simulink model "VehCtrl20260630_18B"  (R2018b)
settings: Solver=FixedStepAuto  StartTime=0.0  StopTime=inf  FixedStep=0.005  RelTol=1e-3
InitFcn:
  | mbd_mpc_consistency_checks(bdroot(gcs));
undefined symbols (not defined in the file): ANG_DEAD, BMS_NormalPwr, BrakeDeadZone, BrkPrsByBrkPct_TB_X, BrkPrsByBrkPct_TB_Y, DELAY_DISCHARGE, DELAY_RCUOFF, DRV_BACKWARD, DRV_BRAKE, DRV_FORWARD, DRV_NEUTRAL, DRV_PARK, DRV_UNPARK, DRV_ZEROTURN, EPB_LOCK, EPB_UNLOCK, ExtraLoadPwr, FanOff, fifo_0_vect, fifo_1_vect, HiFanReq, HV_finished, HV_No_Active, HV_POWER_OFF, HV_POWER_ON, HVDown, HVON, KaTLS_v_DrgUp_X_VehSpd, KeFTM_s_Way1OffDlyTime, KeFTM_TK_Way1CoolLv2OffBatTemp, KeFTM_TK_Way1CoolLv2OffMtrTemp, KeFTM_TK_Way1CoolLv2OnBatTemp, KeFTM_TK_Way1CoolLv2OnMtrTemp, KeFTM_TK_Way1CoolLv3OffBatTemp, KeFTM_TK_Way1CoolLv3OffMtrTemp, KeFTM_TK_Way1CoolLv3OnBatTemp, KeFTM_TK_Way1CoolLv3OnMtrTemp, KeFTM_TK_Way1CoolLv4OffBatTemp, KeFTM_TK_Way1CoolLv4OffMtrTemp, KeFTM_TK_Way1CoolLv4OnBatTemp, KeFTM_TK_Way1CoolLv4OnMtrTemp, Kp1, Kp2, LowFanReq, LQFP, MtrCmdGainFL, MtrCmdGainFR, MtrCmdGainRL, MtrCmdGainRR, MtrPwrFactor_RCU, MtrPwrHighToMidThd, MtrPwrLowToMidThd, MtrPwrMidToHighThd, MtrPwrMidToLowThd, MtrTrqMax, PCT_DEAD, Precharge, PTO_1000, PTO_540, pts1_fifo_0_vect ... (+32)
libraries: mbd_mpc574x_ec_toolbox x175, simulink x110, canmsglib x70
(part 14 of 15)

== system VehCtrl20260630_18B/SigIn/CAN0/AUTO2/UNPACK/Subsystem ==
  In1 : Inport
  CAN_Msg_In : Inport  Port=2
  Action Port : ActionPort  ActionType=else
  Bus Creator1 : BusCreator  Inputs=9
  CAN Unpack6 : canmsglib/CAN Unpack  CANdbFile=E:\硕士工作\0.本周工作\20260428_changchun\VCU_AgriculturalMachinery_260428_ChangChun\VCU_AgriculturalMachinery_260428_ChangChun\CAN协议9.1\AUTO\TractorAuto_Intel.dbc  MsgList=AUTO2VCU_2  MsgName=AUTO2VCU_2  MsgIDType=Extended (29-bit identifier)  MsgIdentifier=4098  MsgLength=8  SignalInfo=AUTO_CheckSum2$56$8$1$2$1$0$1$0$0$255$#AUTO_LiveCnt2$52$4$1$2$1$0$1$0$0$15$#AUTO_PtoSpd$0$16$1$2$1$0$1.000000e-01$-3000$-3000$3000$#AUTO_Shutdown$18$1$1$2$1$0$1$0$0$1$#AUTO_SuspMode$16$2$1$2$1$0$1$0$0$3$#AUTO_Valve1$19$1$1$2$1$0$1$0$0$1$#AUTO_Valve2$20$1$1$2$1$0$1$0$0$1$#AUTO_Valve3$21$1$1$2$1$0$1$0$0$1$#AUTO_Valve4$22$1$1$2$1$0$1$0$0$1$#  NSignals=9  IDPort=off  TimestampPort=off  ErrorPort=off  RemotePort=off  LengthPort=off  StatusPort=off  StartBits=str2num('[int32(56);int32(52);int32(0);int32(18);int32(16);int32(19);int32(20);int32(21);int32(22)]')  SignalSizes=str2num('[int32(8);int32(4);int32(16);int32(1);int32(2);int32(1);int32(1);int32(1);int32(1)]')  ByteOrders=str2num('[int32(1);int32(1);int32(1);int32(1);int32(1);int32(1);int32(1);int32(1);int32(1)]')  DataTypes=str2num('[int32(2);int32(2);int32(2);int32(2);int32(2);int32(2);int32(2);int32(2);int32(2)]')  MultiplexTypes=str2num('[int32(1);int32(1);int32(1);int32(1);int32(1);int32(1);int32(1);int32(1);int32(1)]')  MultiplexValues=str2num('[double(0);double(0);double(0);double(0);double(0);double(0);double(0);double(0);double(0)]')  Factors=str2num('[double(1);double(1);double(1.000000e-01);double(1);double(1);double(1);double(1);double(1);double(1)]')  Offsets=str2num('[double(0);double(0);double(-3000);double(0);double(0);double(0);double(0);double(0);double(0)]')  Minimums=str2num('[double(0);double(0);double(-3000);double(0);double(0);double(0);double(0);double(0);double(0)]')  Maximums=str2num('[double(255);double(15);double(3000);double(1);double(3);double(1);double(1);double(1);double(1)]')  ApplyMinMax=off
      settings: SourceProductName=Simulink Real-Time  SourceProductBaseCode=XP  DataFormat=CANdb specified signals
  Data Type Conversion1 : DataTypeConversion  OutDataTypeStr=uint8
  Data Type Conversion{2..7} (6 alike) : DataTypeConversion  OutDataTypeStr=boolean
  Data Type Conversion61 : DataTypeConversion  OutDataTypeStr=uint8
  Data Type Conversion62 : DataTypeConversion  OutDataTypeStr=single
  Terminator : Terminator
  Out1 : Outport
  wires:
  Data Type Conversion4/1 -> Bus Creator1/1  "AUTO_CheckSum2"
  Data Type Conversion61/1 -> Bus Creator1/2  "AUTO_LiveCnt2"
  Data Type Conversion6/1 -> Bus Creator1/8  "AUTO_Valve3"
  Data Type Conversion3/1 -> Bus Creator1/6  "AUTO_Valve1"
  CAN Unpack6/2 -> Data Type Conversion61/1
  CAN Unpack6/6 -> Data Type Conversion3/1
  CAN Unpack6/3 -> Data Type Conversion62/1
  CAN Unpack6/9 -> Data Type Conversion7/1
  Data Type Conversion62/1 -> Bus Creator1/3  "AUTO_PtoSpd"
  Data Type Conversion5/1 -> Bus Creator1/7  "AUTO_Valve2"
  Data Type Conversion1/1 -> Bus Creator1/5  "AUTO_SuspMode"
  Data Type Conversion2/1 -> Bus Creator1/4  "AUTO_Shutdown"
  Bus Creator1/1 -> Out1/1
  CAN Unpack6/8 -> Data Type Conversion6/1
  CAN Unpack6/5 -> Data Type Conversion1/1
  CAN Unpack6/4 -> Data Type Conversion2/1
  Data Type Conversion7/1 -> Bus Creator1/9  "AUTO_Valve4"
  CAN Unpack6/7 -> Data Type Conversion5/1
  CAN_Msg_In/1 -> CAN Unpack6/1
  CAN Unpack6/1 -> Terminator/1
  In1/1 -> Data Type Conversion4/1

== system VehCtrl20260630_18B/SigIn/CAN0/AUTO3/UNPACK/If Action Subsystem ==
  In1 : Inport
  Action Port : ActionPort  ActionType=then
  Out1 : Outport
  wires:
  In1/1 -> Out1/1

== system VehCtrl20260630_18B/SigIn/CAN0/AUTO3/UNPACK/Subsystem ==
  In1 : Inport
  CAN_Msg_In : Inport  Port=2
  Action Port : ActionPort  ActionType=else
  Bus Creator1 : BusCreator  Inputs=6
  CAN Unpack6 : canmsglib/CAN Unpack  CANdbFile=E:\硕士工作\0.本周工作\20260428_changchun\VCU_260508_ChangChun\CAN协议0509\AUTO\TractorAuto_Intel0511.dbc  MsgList=AUTO2VCU_3  MsgName=AUTO2VCU_3  MsgIDType=Extended (29-bit identifier)  MsgIdentifier=4099  MsgLength=8  SignalInfo=AUTO_CheckSum3$56$8$1$2$1$0$1$0$0$255$#AUTO_LiveCnt3$52$4$1$2$1$0$1$0$0$15$#TrqCmdFL$0$12$1$2$1$0$1.000000e-01$-200$-200$200$#TrqCmdFR$12$12$1$2$1$0$1.000000e-01$-200$-200$200$#TrqCmdRL$24$12$1$2$1$0$1.000000e-01$-200$-200$200$#TrqCmdRR$36$12$1$2$1$0$1.000000e-01$-200$-200$200$#  NSignals=6  IDPort=off  TimestampPort=off  ErrorPort=off  RemotePort=off  LengthPort=off  StatusPort=off  StartBits=str2num('[int32(56);int32(52);int32(0);int32(12);int32(24);int32(36)]')  SignalSizes=str2num('[int32(8);int32(4);int32(12);int32(12);int32(12);int32(12)]')  ByteOrders=str2num('[int32(1);int32(1);int32(1);int32(1);int32(1);int32(1)]')  DataTypes=str2num('[int32(2);int32(2);int32(2);int32(2);int32(2);int32(2)]')  MultiplexTypes=str2num('[int32(1);int32(1);int32(1);int32(1);int32(1);int32(1)]')  MultiplexValues=str2num('[double(0);double(0);double(0);double(0);double(0);double(0)]')  Factors=str2num('[double(1);double(1);double(1.000000e-01);double(1.000000e-01);double(1.000000e-01);double(1.000000e-01)]')  Offsets=str2num('[double(0);double(0);double(-200);double(-200);double(-200);double(-200)]')  Minimums=str2num('[double(0);double(0);double(-200);double(-200);double(-200);double(-200)]')  Maximums=str2num('[double(255);double(15);double(200);double(200);double(200);double(200)]')  ApplyMinMax=off
      settings: SourceProductName=Simulink Real-Time  SourceProductBaseCode=XP  DataFormat=CANdb specified signals
  Data Type Conversion{1,3..5} (4 alike) : DataTypeConversion  OutDataTypeStr=single
  Data Type Conversion2 : DataTypeConversion  OutDataTypeStr=uint8
  Data Type Conversion61 : DataTypeConversion  OutDataTypeStr=boolean
  Terminator1 : Terminator
  Out1 : Outport
  wires:
  In1/1 -> Data Type Conversion61/1
  CAN_Msg_In/1 -> CAN Unpack6/1
  Bus Creator1/1 -> Out1/1
  Data Type Conversion3/1 -> Bus Creator1/4  "AUTO_TrqCmdFR"
  Data Type Conversion1/1 -> Bus Creator1/3  "AUTO_TrqCmdFL"
  Data Type Conversion5/1 -> Bus Creator1/5  "AUTO_TrqCmdRL"
  Data Type Conversion2/1 -> Bus Creator1/2  "AUTO_LiveCnt1"
  Data Type Conversion61/1 -> Bus Creator1/1  "AUTO_CheckSum1"
  CAN Unpack6/1 -> Terminator1/1
  CAN Unpack6/2 -> Data Type Conversion2/1
  Data Type Conversion4/1 -> Bus Creator1/6  "AUTO_TrqCmdRR"
  CAN Unpack6/3 -> Data Type Conversion1/1
  CAN Unpack6/4 -> Data Type Conversion3/1
  CAN Unpack6/5 -> Data Type Conversion5/1
  CAN Unpack6/6 -> Data Type Conversion4/1

== system VehCtrl20260630_18B/SigIn/CAN0/RMT_VCU1/UNPACK/Subsystem ==
  In1 : Inport
  Add : Sum  Inputs=+-
  Constant : Constant  Value=1000  OutDataTypeStr=single
  Gain : Gain  Gain=100/666
  Saturation : Saturate  UpperLimit=100  LowerLimit=0
  Out1 : Outport
  wires:
  Add/1 -> Gain/1
  Constant/1 -> Add/1
  In1/1 -> Add/2
  Gain/1 -> Saturation/1
  Saturation/1 -> Out1/1

== system VehCtrl20260630_18B/SigIn/CAN0/RMT_VCU1/UNPACK/Subsystem1 ==
  In1 : Inport
  Add : Sum  Inputs=+-
  Constant : Constant  Value=1000  OutDataTypeStr=single
  Gain : Gain  Gain=100/666
  Gain1 : Gain  Gain=-1
  Saturation : Saturate  UpperLimit=100  LowerLimit=0
  Out1 : Outport
  wires:
  Saturation/1 -> Out1/1
  Gain/1 -> Gain1/1
  In1/1 -> Add/2
  Constant/1 -> Add/1
  Add/1 -> Gain/1
  Gain1/1 -> Saturation/1

== system VehCtrl20260630_18B/SigIn/CAN0/RMT_VCU1/UNPACK/Subsystem2 ==
  In1 : Inport
  Add : Sum  Inputs=+-
  Constant : Constant  Value=1000  OutDataTypeStr=single
  Gain : Gain  Gain=45/666
  Out1 : Outport
  wires:
  Add/1 -> Gain/1
  Constant/1 -> Add/1
  In1/1 -> Add/2
  Gain/1 -> Out1/1

== system VehCtrl20260630_18B/SigIn/CAN0/RMT_VCU2/UNPACK/Subsystem ==
  RMT_MtrTqGr : Inport
  Add1 : Sum  Inputs=+-
  Constant2 : Constant  Value=333  OutDataTypeStr=single
  Gain : Gain  Gain=1/1333
  Saturation : Saturate  UpperLimit=1  LowerLimit=0
  Out1 : Outport
  wires:
  Constant2/1 -> Add1/2
  Add1/1 -> Gain/1
  Saturation/1 -> Out1/1
  Gain/1 -> Saturation/1
  RMT_MtrTqGr/1 -> Add1/1

== system VehCtrl20260630_18B/SigIn/CAN0/RMT_VCU2/UNPACK/Subsystem3 ==
  In1 : Inport
  Constant2 : Constant  Value=1350  OutDataTypeStr=single
  Constant3 : Constant  Value=650  OutDataTypeStr=single
  Constant6 : Constant  Value=2  OutDataTypeStr=uint8
  Constant7 : Constant  OutDataTypeStr=uint8
  Constant8 : Constant  Value=0  OutDataTypeStr=uint8
  Data Type Conversion4 : DataTypeConversion  OutDataTypeStr=single
  GreaterThan : RelationalOperator  Operator=>  OutDataTypeStr=boolean  RndMeth=Simplest
  GreaterThan1 : RelationalOperator  Operator=<  OutDataTypeStr=boolean  RndMeth=Simplest
  Switch : Switch  Criteria=u2 > Threshold
  Switch1 : Switch  Criteria=u2 > Threshold
  Out1 : Outport
  wires:
  In1/1 -> Data Type Conversion4/1
  GreaterThan1/1 -> Switch1/2
  Constant6/1 -> Switch/1
  GreaterThan/1 -> Switch/2
  Constant7/1 -> Switch1/1
  Data Type Conversion4/1 -> GreaterThan1/1, GreaterThan/1
  Switch/1 -> Out1/1
  Switch1/1 -> Switch/3
  Constant3/1 -> GreaterThan1/2
  Constant2/1 -> GreaterThan/2
  Constant8/1 -> Switch1/3

== system VehCtrl20260630_18B/SigIn/CAN0/RMT_VCU2/UNPACK/Subsystem4 ==
  In1 : Inport
  Constant2 : Constant  Value=1350  OutDataTypeStr=single
  Constant3 : Constant  Value=650  OutDataTypeStr=single
  Constant6 : Constant  OutDataTypeStr=uint8
  Constant7 : Constant  Value=2  OutDataTypeStr=uint8
  Constant8 : Constant  Value=0  OutDataTypeStr=uint8
  Data Type Conversion4 : DataTypeConversion  OutDataTypeStr=single
  GreaterThan : RelationalOperator  Operator=>  OutDataTypeStr=boolean  RndMeth=Simplest
  GreaterThan1 : RelationalOperator  Operator=<  OutDataTypeStr=boolean  RndMeth=Simplest
  Switch : Switch  Criteria=u2 > Threshold
  Switch1 : Switch  Criteria=u2 > Threshold
  Out1 : Outport
  wires:
  In1/1 -> Data Type Conversion4/1
  GreaterThan1/1 -> Switch1/2
  Constant6/1 -> Switch/1
  GreaterThan/1 -> Switch/2
  Constant7/1 -> Switch1/1
  Data Type Conversion4/1 -> GreaterThan1/1, GreaterThan/1
  Switch/1 -> Out1/1
  Switch1/1 -> Switch/3
  Constant3/1 -> GreaterThan1/2
  Constant2/1 -> GreaterThan/2
  Constant8/1 -> Switch1/3

== system VehCtrl20260630_18B/SigIn/CAN0/RMT_VCU3/UNPACK/Subsystem1 ==
  In1 : Inport
  Constant1 : Constant  Value=1200  OutDataTypeStr=single
  Constant3 : Constant  OutDataTypeStr=uint8
  Constant4 : Constant  Value=0  OutDataTypeStr=uint8
  GreaterThan1 : RelationalOperator  OutDataTypeStr=boolean  RndMeth=Simplest
  Switch1 : Switch  Criteria=u2 > Threshold
  Out1 : Outport
  wires:
  Switch1/1 -> Out1/1
  In1/1 -> GreaterThan1/1
  Constant1/1 -> GreaterThan1/2
  GreaterThan1/1 -> Switch1/2
  Constant3/1 -> Switch1/1
  Constant4/1 -> Switch1/3

== system VehCtrl20260630_18B/SigIn/CAN0/RMT_VCU3/UNPACK/Subsystem2 ==
  In1 : Inport
  Constant1 : Constant  Value=800  OutDataTypeStr=single
  Constant3 : Constant  OutDataTypeStr=uint8
  Constant4 : Constant  Value=0  OutDataTypeStr=uint8
  Data Type Conversion : DataTypeConversion  OutDataTypeStr=single
  Data Type Conversion2 : DataTypeConversion  OutDataTypeStr=boolean
  GreaterThan1 : RelationalOperator  Operator=<  OutDataTypeStr=boolean  RndMeth=Simplest
  Switch1 : Switch  Criteria=u2 > Threshold
  Out1 : Outport
  wires:
  Constant4/1 -> Switch1/3
  Constant3/1 -> Switch1/1
  GreaterThan1/1 -> Switch1/2
  Constant1/1 -> GreaterThan1/2
  Data Type Conversion/1 -> GreaterThan1/1
  In1/1 -> Data Type Conversion/1
  Switch1/1 -> Data Type Conversion2/1
  Data Type Conversion2/1 -> Out1/1  "RMT_Auto"

== system VehCtrl20260630_18B/SigIn/CAN0/RMT_VCU3/UNPACK/Subsystem4 ==
  In1 : Inport
  Constant1 : Constant  Value=1200  OutDataTypeStr=single
  Constant3 : Constant  OutDataTypeStr=uint8
  Constant4 : Constant  Value=0  OutDataTypeStr=uint8
  GreaterThan1 : RelationalOperator  Operator=>  OutDataTypeStr=boolean  RndMeth=Simplest
  Switch1 : Switch  Criteria=u2 > Threshold
  Out1 : Outport
  wires:
  Constant4/1 -> Switch1/3
  Constant3/1 -> Switch1/1
  GreaterThan1/1 -> Switch1/2
  Constant1/1 -> GreaterThan1/2
  In1/1 -> GreaterThan1/1
  Switch1/1 -> Out1/1

== system VehCtrl20260630_18B/SigIn/CAN0/RMT_VCU3/UNPACK/Subsystem5 ==
  In1 : Inport
  Constant1 : Constant  Value=800  OutDataTypeStr=single
  Constant3 : Constant  OutDataTypeStr=uint8
  Constant4 : Constant  Value=0  OutDataTypeStr=uint8
  Data Type Conversion : DataTypeConversion  OutDataTypeStr=single
  GreaterThan1 : RelationalOperator  Operator=<  OutDataTypeStr=boolean  RndMeth=Simplest
  Switch1 : Switch  Criteria=u2 > Threshold
  Out1 : Outport
  wires:
  Switch1/1 -> Out1/1
  In1/1 -> Data Type Conversion/1
  Data Type Conversion/1 -> GreaterThan1/1
  Constant1/1 -> GreaterThan1/2
  GreaterThan1/1 -> Switch1/2
  Constant3/1 -> Switch1/1
  Constant4/1 -> Switch1/3

== system VehCtrl20260630_18B/SigIn/CAN0/RMT_VCU4/UNPACK/Subsystem1 ==
  In1 : Inport
  Constant : Constant  Value=1200  OutDataTypeStr=single
  Constant1 : Constant  Value=800  OutDataTypeStr=single
  Constant2 : Constant  Value=2  OutDataTypeStr=uint8
  Constant3 : Constant  OutDataTypeStr=uint8
  Constant4 : Constant  Value=0  OutDataTypeStr=uint8
  Data Type Conversion : DataTypeConversion  OutDataTypeStr=single
  GreaterThan : RelationalOperator  Operator=>  OutDataTypeStr=boolean  RndMeth=Simplest
  GreaterThan1 : RelationalOperator  Operator=<  OutDataTypeStr=boolean  RndMeth=Simplest
  Switch : Switch  Criteria=u2 > Threshold
  Switch1 : Switch  Criteria=u2 > Threshold
  Out1 : Outport
  wires:
  Constant4/1 -> Switch1/3
  Constant3/1 -> Switch1/1
  Constant2/1 -> Switch/1
  Switch/1 -> Out1/1
  Switch1/1 -> Switch/3
  GreaterThan1/1 -> Switch1/2
  GreaterThan/1 -> Switch/2
  Constant1/1 -> GreaterThan1/2
  Data Type Conversion/1 -> GreaterThan/1, GreaterThan1/1
  Constant/1 -> GreaterThan/2
  In1/1 -> Data Type Conversion/1

== system VehCtrl20260630_18B/SigIn/CAN0/RMT_VCU4/UNPACK/Subsystem2 ==
  In1 : Inport
  Constant : Constant  Value=1200  OutDataTypeStr=single
  Constant1 : Constant  Value=800  OutDataTypeStr=single
  Constant2 : Constant  Value=2  OutDataTypeStr=uint8
  Constant3 : Constant  OutDataTypeStr=uint8
  Constant4 : Constant  Value=0  OutDataTypeStr=uint8
  Data Type Conversion : DataTypeConversion  OutDataTypeStr=single
  GreaterThan : RelationalOperator  Operator=>  OutDataTypeStr=boolean  RndMeth=Simplest
  GreaterThan1 : RelationalOperator  Operator=<  OutDataTypeStr=boolean  RndMeth=Simplest
  Switch : Switch  Criteria=u2 > Threshold
  Switch1 : Switch  Criteria=u2 > Threshold
  Out1 : Outport
  wires:
  In1/1 -> Data Type Conversion/1
  Constant/1 -> GreaterThan/2
  Data Type Conversion/1 -> GreaterThan1/1, GreaterThan/1
  Constant1/1 -> GreaterThan1/2
  GreaterThan/1 -> Switch/2
  GreaterThan1/1 -> Switch1/2
  Switch1/1 -> Switch/3
  Switch/1 -> Out1/1
  Constant2/1 -> Switch/1
  Constant3/1 -> Switch1/1
  Constant4/1 -> Switch1/3

== system VehCtrl20260630_18B/SigIn/CAN0/RMT_VCU4/UNPACK/Subsystem3 ==
  In1 : Inport
  Constant1 : Constant  Value=800  OutDataTypeStr=single
  Constant3 : Constant  OutDataTypeStr=uint8
  Constant4 : Constant  Value=0  OutDataTypeStr=uint8
  Data Type Conversion : DataTypeConversion  OutDataTypeStr=single
  GreaterThan1 : RelationalOperator  Operator=<  OutDataTypeStr=boolean  RndMeth=Simplest
  Switch1 : Switch  Criteria=u2 > Threshold
  Out1 : Outport
  wires:
  Constant4/1 -> Switch1/3
  Constant3/1 -> Switch1/1
  GreaterThan1/1 -> Switch1/2
  Constant1/1 -> GreaterThan1/2
  Data Type Conversion/1 -> GreaterThan1/1
  In1/1 -> Data Type Conversion/1
  Switch1/1 -> Out1/1

== system VehCtrl20260630_18B/SigIn/CAN0/RMT_VCU4/UNPACK/Subsystem4 ==
  In1 : Inport
  Constant1 : Constant  Value=800  OutDataTypeStr=single
  Constant3 : Constant  OutDataTypeStr=uint8
  Constant4 : Constant  Value=0  OutDataTypeStr=uint8
  Data Type Conversion : DataTypeConversion  OutDataTypeStr=single
  GreaterThan1 : RelationalOperator  Operator=<  OutDataTypeStr=boolean  RndMeth=Simplest
  Switch1 : Switch  Criteria=u2 > Threshold
  Out1 : Outport
  wires:
  Switch1/1 -> Out1/1
  In1/1 -> Data Type Conversion/1
  Data Type Conversion/1 -> GreaterThan1/1
  Constant1/1 -> GreaterThan1/2
  GreaterThan1/1 -> Switch1/2
  Constant3/1 -> Switch1/1
  Constant4/1 -> Switch1/3

== system VehCtrl20260630_18B/SigIn/CAN1/MCU2VCU_1/UNPACK/Subsystem ==
  WorkStatus : Inport
  Bitwise Operator : simulink/Logic and Bit Operations/Bitwise Operator  logicop=AND  UseBitMask=on  BitMask=bin2dec('00000001')  BitMaskRealWorld=Stored Integer
  Bitwise Operator1 : simulink/Logic and Bit Operations/Bitwise Operator  logicop=AND  UseBitMask=on  BitMask=bin2dec('00000010')  BitMaskRealWorld=Stored Integer
  Bitwise Operator2 : simulink/Logic and Bit Operations/Bitwise Operator  logicop=AND  UseBitMask=on  BitMask=bin2dec('00000100')  BitMaskRealWorld=Stored Integer
  Bitwise Operator3 : simulink/Logic and Bit Operations/Bitwise Operator  logicop=AND  UseBitMask=on  BitMask=bin2dec('00001000')  BitMaskRealWorld=Stored Integer
  Bitwise Operator4 : simulink/Logic and Bit Operations/Bitwise Operator  logicop=AND  UseBitMask=on  BitMask=bin2dec('00010000')  BitMaskRealWorld=Stored Integer
  Bitwise Operator5 : simulink/Logic and Bit Operations/Bitwise Operator  logicop=AND  UseBitMask=on  BitMask=bin2dec('00100000')  BitMaskRealWorld=Stored Integer
  Bitwise Operator6 : simulink/Logic and Bit Operations/Bitwise Operator  logicop=AND  UseBitMask=on  BitMask=bin2dec('01000000')  BitMaskRealWorld=Stored Integer
  Bitwise Operator7 : simulink/Logic and Bit Operations/Bitwise Operator  logicop=AND  UseBitMask=on  BitMask=bin2dec('10000000')  BitMaskRealWorld=Stored Integer
  NOT : Logic  Operator=NOT  IconShape=distinctive  AllPortsSameDT=off  OutDataTypeStr=boolean
  StartORStop : Outport
  Discharge : Outport  Port=2
  Direction : Outport  Port=3
  DrvORBrk : Outport  Port=4
  Fault : Outport  Port=5
  Ready : Outport  Port=6
  Mode : Outport  Port=7
  PWM : Outport  Port=8
  wires:
  WorkStatus/1 -> Bitwise Operator7/1, Bitwise Operator6/1, Bitwise Operator5/1, Bitwise Operator4/1, Bitwise Operator3/1, Bitwise Operator2/1, Bitwise Operator1/1, Bitwise Operator/1
  Bitwise Operator/1 -> StartORStop/1
  Bitwise Operator1/1 -> Discharge/1
  Bitwise Operator2/1 -> NOT/1
  Bitwise Operator5/1 -> Ready/1
  Bitwise Operator4/1 -> Fault/1
  Bitwise Operator3/1 -> DrvORBrk/1
  Bitwise Operator6/1 -> Mode/1
  Bitwise Operator7/1 -> PWM/1
  NOT/1 -> Direction/1

== system VehCtrl20260630_18B/SigIn/CAN1/MCU2VCU_13/UNPACK/Subsystem ==
  WorkStatus : Inport
  Bitwise Operator : simulink/Logic and Bit Operations/Bitwise Operator  logicop=AND  UseBitMask=on  BitMask=bin2dec('00000001')  BitMaskRealWorld=Stored Integer
  Bitwise Operator1 : simulink/Logic and Bit Operations/Bitwise Operator  logicop=AND  UseBitMask=on  BitMask=bin2dec('00000010')  BitMaskRealWorld=Stored Integer
  Bitwise Operator2 : simulink/Logic and Bit Operations/Bitwise Operator  logicop=AND  UseBitMask=on  BitMask=bin2dec('00000100')  BitMaskRealWorld=Stored Integer
  Bitwise Operator3 : simulink/Logic and Bit Operations/Bitwise Operator  logicop=AND  UseBitMask=on  BitMask=bin2dec('00001000')  BitMaskRealWorld=Stored Integer
  Bitwise Operator4 : simulink/Logic and Bit Operations/Bitwise Operator  logicop=AND  UseBitMask=on  BitMask=bin2dec('00010000')  BitMaskRealWorld=Stored Integer
  Bitwise Operator5 : simulink/Logic and Bit Operations/Bitwise Operator  logicop=AND  UseBitMask=on  BitMask=bin2dec('00100000')  BitMaskRealWorld=Stored Integer
  Bitwise Operator6 : simulink/Logic and Bit Operations/Bitwise Operator  logicop=AND  UseBitMask=on  BitMask=bin2dec('01000000')  BitMaskRealWorld=Stored Integer
  Bitwise Operator7 : simulink/Logic and Bit Operations/Bitwise Operator  logicop=AND  UseBitMask=on  BitMask=bin2dec('10000000')  BitMaskRealWorld=Stored Integer
  NOT : Logic  Operator=NOT  IconShape=distinctive  AllPortsSameDT=off  OutDataTypeStr=boolean
  StartORStop : Outport
  Discharge : Outport  Port=2
  Direction : Outport  Port=3
  DrvORBrk : Outport  Port=4
  Fault : Outport  Port=5
  Ready : Outport  Port=6
  Mode : Outport  Port=7
  PWM : Outport  Port=8
  wires:
  WorkStatus/1 -> Bitwise Operator7/1, Bitwise Operator6/1, Bitwise Operator5/1, Bitwise Operator4/1, Bitwise Operator3/1, Bitwise Operator2/1, Bitwise Operator1/1, Bitwise Operator/1
  Bitwise Operator/1 -> StartORStop/1
  Bitwise Operator1/1 -> Discharge/1
  Bitwise Operator2/1 -> NOT/1
  Bitwise Operator5/1 -> Ready/1
  Bitwise Operator4/1 -> Fault/1
  Bitwise Operator3/1 -> DrvORBrk/1
  Bitwise Operator6/1 -> Mode/1
  Bitwise Operator7/1 -> PWM/1
  NOT/1 -> Direction/1

== system VehCtrl20260630_18B/SigIn/CAN1/MCU2VCU_17/UNPACK/Subsystem ==
  WorkStatus : Inport
  Bitwise Operator : simulink/Logic and Bit Operations/Bitwise Operator  logicop=AND  UseBitMask=on  BitMask=bin2dec('00000001')  BitMaskRealWorld=Stored Integer
  Bitwise Operator1 : simulink/Logic and Bit Operations/Bitwise Operator  logicop=AND  UseBitMask=on  BitMask=bin2dec('00000010')  BitMaskRealWorld=Stored Integer
  Bitwise Operator2 : simulink/Logic and Bit Operations/Bitwise Operator  logicop=AND  UseBitMask=on  BitMask=bin2dec('00000100')  BitMaskRealWorld=Stored Integer
  Bitwise Operator3 : simulink/Logic and Bit Operations/Bitwise Operator  logicop=AND  UseBitMask=on  BitMask=bin2dec('00001000')  BitMaskRealWorld=Stored Integer
  Bitwise Operator4 : simulink/Logic and Bit Operations/Bitwise Operator  logicop=AND  UseBitMask=on  BitMask=bin2dec('00010000')  BitMaskRealWorld=Stored Integer
  Bitwise Operator5 : simulink/Logic and Bit Operations/Bitwise Operator  logicop=AND  UseBitMask=on  BitMask=bin2dec('00100000')  BitMaskRealWorld=Stored Integer
  Bitwise Operator6 : simulink/Logic and Bit Operations/Bitwise Operator  logicop=AND  UseBitMask=on  BitMask=bin2dec('01000000')  BitMaskRealWorld=Stored Integer
  Bitwise Operator7 : simulink/Logic and Bit Operations/Bitwise Operator  logicop=AND  UseBitMask=on  BitMask=bin2dec('10000000')  BitMaskRealWorld=Stored Integer
  NOT : Logic  Operator=NOT  IconShape=distinctive  AllPortsSameDT=off  OutDataTypeStr=boolean
  StartORStop : Outport
  Discharge : Outport  Port=2
  Direction : Outport  Port=3
  DrvORBrk : Outport  Port=4
  Fault : Outport  Port=5
  Ready : Outport  Port=6
  Mode : Outport  Port=7
  PWM : Outport  Port=8
  wires:
  WorkStatus/1 -> Bitwise Operator7/1, Bitwise Operator6/1, Bitwise Operator5/1, Bitwise Operator4/1, Bitwise Operator3/1, Bitwise Operator2/1, Bitwise Operator1/1, Bitwise Operator/1
  Bitwise Operator/1 -> StartORStop/1
  Bitwise Operator1/1 -> Discharge/1
  Bitwise Operator2/1 -> NOT/1
  Bitwise Operator5/1 -> Ready/1
  Bitwise Operator4/1 -> Fault/1
  Bitwise Operator3/1 -> DrvORBrk/1
  Bitwise Operator6/1 -> Mode/1
  Bitwise Operator7/1 -> PWM/1
  NOT/1 -> Direction/1

== system VehCtrl20260630_18B/SigIn/CAN1/MCU2VCU_5/UNPACK/Subsystem ==
  WorkStatus : Inport
  Bitwise Operator : simulink/Logic and Bit Operations/Bitwise Operator  logicop=AND  UseBitMask=on  BitMask=bin2dec('00000001')  BitMaskRealWorld=Stored Integer
  Bitwise Operator1 : simulink/Logic and Bit Operations/Bitwise Operator  logicop=AND  UseBitMask=on  BitMask=bin2dec('00000010')  BitMaskRealWorld=Stored Integer
  Bitwise Operator2 : simulink/Logic and Bit Operations/Bitwise Operator  logicop=AND  UseBitMask=on  BitMask=bin2dec('00000100')  BitMaskRealWorld=Stored Integer
  Bitwise Operator3 : simulink/Logic and Bit Operations/Bitwise Operator  logicop=AND  UseBitMask=on  BitMask=bin2dec('00001000')  BitMaskRealWorld=Stored Integer
  Bitwise Operator4 : simulink/Logic and Bit Operations/Bitwise Operator  logicop=AND  UseBitMask=on  BitMask=bin2dec('00010000')  BitMaskRealWorld=Stored Integer
  Bitwise Operator5 : simulink/Logic and Bit Operations/Bitwise Operator  logicop=AND  UseBitMask=on  BitMask=bin2dec('00100000')  BitMaskRealWorld=Stored Integer
  Bitwise Operator6 : simulink/Logic and Bit Operations/Bitwise Operator  logicop=AND  UseBitMask=on  BitMask=bin2dec('01000000')  BitMaskRealWorld=Stored Integer
  Bitwise Operator7 : simulink/Logic and Bit Operations/Bitwise Operator  logicop=AND  UseBitMask=on  BitMask=bin2dec('10000000')  BitMaskRealWorld=Stored Integer
  StartORStop : Outport
  Discharge : Outport  Port=2
  Direction : Outport  Port=3
  DrvORBrk : Outport  Port=4
  Fault : Outport  Port=5
  Ready : Outport  Port=6
  Mode : Outport  Port=7
  PWM : Outport  Port=8
  wires:
  WorkStatus/1 -> Bitwise Operator7/1, Bitwise Operator6/1, Bitwise Operator5/1, Bitwise Operator4/1, Bitwise Operator3/1, Bitwise Operator2/1, Bitwise Operator1/1, Bitwise Operator/1
  Bitwise Operator/1 -> StartORStop/1
  Bitwise Operator1/1 -> Discharge/1
  Bitwise Operator5/1 -> Ready/1
  Bitwise Operator4/1 -> Fault/1
  Bitwise Operator3/1 -> DrvORBrk/1
  Bitwise Operator6/1 -> Mode/1
  Bitwise Operator7/1 -> PWM/1
  Bitwise Operator2/1 -> Direction/1

== system VehCtrl20260630_18B/SigIn/CAN1/MCU2VCU_9/UNPACK/Subsystem ==
  WorkStatus : Inport
  Bitwise Operator : simulink/Logic and Bit Operations/Bitwise Operator  logicop=AND  UseBitMask=on  BitMask=bin2dec('00000001')  BitMaskRealWorld=Stored Integer
  Bitwise Operator1 : simulink/Logic and Bit Operations/Bitwise Operator  logicop=AND  UseBitMask=on  BitMask=bin2dec('00000010')  BitMaskRealWorld=Stored Integer
  Bitwise Operator2 : simulink/Logic and Bit Operations/Bitwise Operator  logicop=AND  UseBitMask=on  BitMask=bin2dec('00000100')  BitMaskRealWorld=Stored Integer
  Bitwise Operator3 : simulink/Logic and Bit Operations/Bitwise Operator  logicop=AND  UseBitMask=on  BitMask=bin2dec('00001000')  BitMaskRealWorld=Stored Integer
  Bitwise Operator4 : simulink/Logic and Bit Operations/Bitwise Operator  logicop=AND  UseBitMask=on  BitMask=bin2dec('00010000')  BitMaskRealWorld=Stored Integer
  Bitwise Operator5 : simulink/Logic and Bit Operations/Bitwise Operator  logicop=AND  UseBitMask=on  BitMask=bin2dec('00100000')  BitMaskRealWorld=Stored Integer
  Bitwise Operator6 : simulink/Logic and Bit Operations/Bitwise Operator  logicop=AND  UseBitMask=on  BitMask=bin2dec('01000000')  BitMaskRealWorld=Stored Integer
  Bitwise Operator7 : simulink/Logic and Bit Operations/Bitwise Operator  logicop=AND  UseBitMask=on  BitMask=bin2dec('10000000')  BitMaskRealWorld=Stored Integer
  NOT : Logic  Operator=NOT  IconShape=distinctive  AllPortsSameDT=off  OutDataTypeStr=boolean
  StartORStop : Outport
  Discharge : Outport  Port=2
  Direction : Outport  Port=3
  DrvORBrk : Outport  Port=4
  Fault : Outport  Port=5
  Ready : Outport  Port=6
  Mode : Outport  Port=7
  PWM : Outport  Port=8
  wires:
  WorkStatus/1 -> Bitwise Operator7/1, Bitwise Operator6/1, Bitwise Operator5/1, Bitwise Operator4/1, Bitwise Operator3/1, Bitwise Operator2/1, Bitwise Operator1/1, Bitwise Operator/1
  Bitwise Operator/1 -> StartORStop/1
  Bitwise Operator1/1 -> Discharge/1
  Bitwise Operator2/1 -> NOT/1
  Bitwise Operator5/1 -> Ready/1
  Bitwise Operator4/1 -> Fault/1
  Bitwise Operator3/1 -> DrvORBrk/1
  Bitwise Operator6/1 -> Mode/1
  Bitwise Operator7/1 -> PWM/1
  NOT/1 -> Direction/1

== system VehCtrl20260630_18B/SigIn/PWM/Subsystem/eTimer Configuration and Signal Measurements/Subsystem_capture ==
  In1 : Inport
  function : TriggerPort  TriggerType=function-call  VariantControl=Variant
  Terminator : Terminator
  eTimer_Arm_Capture : mbd_mpc574x_ec_toolbox/Motor Control Blocks/eTIMER Blocks/eTimer_Arm_Capture  etimerModule=0  etimerChannel=1  etimerArmAction=Stop
  eTimer_Capture : mbd_mpc574x_ec_toolbox/Motor Control Blocks/eTIMER Blocks/eTimer_Capture  etimerModule=0  etimerChannel=1
  Out1 : Outport  OutDataTypeStr=uint16
  Out2 : Outport  Port=2  OutDataTypeStr=uint16
  Out3 : Outport  Port=3  OutDataTypeStr=uint16
  Out4 : Outport  Port=4  OutDataTypeStr=uint16
  wires:
  eTimer_Capture/1 -> Out1/1
  eTimer_Capture/4 -> Out4/1
  eTimer_Capture/3 -> Out3/1
  eTimer_Capture/2 -> Out2/1
  In1/1 -> Terminator/1

== system VehCtrl20260630_18B/SigOut/GPIO /SPI0: LS09_14_15_16_1_2_11_4/LS_CTRL/If Action Subsystem1 ==
  Add : Sum  Inputs=++++
  Constant1 : Constant  Value=128  OutDataTypeStr=uint8
  Constant2 : Constant  Value=64  OutDataTypeStr=uint8
  Constant3 : Constant  Value=32  OutDataTypeStr=uint8
  Constant4 : Constant  Value=16  OutDataTypeStr=uint8
  Constant5 : Constant  Value=8  OutDataTypeStr=uint8
  Constant6 : Constant  Value=4  OutDataTypeStr=uint8
  Constant7 : Constant  Value=2  OutDataTypeStr=uint8
  Constant8 : Constant  OutDataTypeStr=uint8
  Constant9 : Constant  Value=128  OutDataTypeStr=uint8
  Data Store Read : DataStoreRead  DataStoreName=LS004
  Data Store Read4 : DataStoreRead  DataStoreName=LS011
  Data Store Read5 : DataStoreRead  DataStoreName=LS001
  Data Store Read6 : DataStoreRead  DataStoreName=LS002
  Data Type Conversion : DataTypeConversion
  Data Type Conversion1 : DataTypeConversion
  Switch{,1..3} (4 alike) : Switch  Criteria=u2 > Threshold
  Out1 : Outport
  Out2 : Outport  Port=2
  wires:
  Constant2/1 -> Switch/3
  Constant1/1 -> Switch/1
  Add/1 -> Data Type Conversion1/1
  Data Store Read6/1 -> Switch/2
  Constant7/1 -> Switch3/1
  Switch1/1 -> Add/2
  Constant5/1 -> Switch2/1
  Switch/1 -> Add/1
  Constant4/1 -> Switch1/3
  Data Store Read/1 -> Switch3/2
  Switch2/1 -> Add/3
  Data Store Read4/1 -> Switch2/2
  Switch3/1 -> Add/4
  Constant3/1 -> Switch1/1
  Data Store Read5/1 -> Switch1/2
  Constant8/1 -> Switch3/3
  Constant9/1 -> Data Type Conversion/1
  Constant6/1 -> Switch2/3
  Data Type Conversion/1 -> Out1/1
  Data Type Conversion1/1 -> Out2/1

== system VehCtrl20260630_18B/SigOut/GPIO /SPI0: LS09_14_15_16_1_2_11_4/LS_CTRL1/If Action Subsystem1 ==
  Add : Sum  Inputs=++++
  Constant1 : Constant  Value=128  OutDataTypeStr=uint8
  Constant2 : Constant  Value=64  OutDataTypeStr=uint8
  Constant3 : Constant  Value=32  OutDataTypeStr=uint8
  Constant4 : Constant  Value=16  OutDataTypeStr=uint8
  Constant5 : Constant  Value=8  OutDataTypeStr=uint8
  Constant6 : Constant  Value=4  OutDataTypeStr=uint8
  Constant7 : Constant  Value=2  OutDataTypeStr=uint8
  Constant8 : Constant  OutDataTypeStr=uint8
  Constant9 : Constant  Value=128  OutDataTypeStr=uint8
  Data Store Read : DataStoreRead  DataStoreName=LS014
  Data Store Read4 : DataStoreRead  DataStoreName=LS015
  Data Store Read5 : DataStoreRead  DataStoreName=LS009
  Data Store Read6 : DataStoreRead  DataStoreName=LS016
  Data Type Conversion : DataTypeConversion
  Data Type Conversion1 : DataTypeConversion
  Switch{,1..3} (4 alike) : Switch  Criteria=u2 > Threshold
  Out1 : Outport
  Out2 : Outport  Port=2
  wires:
  Data Type Conversion1/1 -> Out2/1
  Data Type Conversion/1 -> Out1/1
  Constant6/1 -> Switch2/3
  Constant9/1 -> Data Type Conversion/1
  Constant8/1 -> Switch3/3
  Data Store Read5/1 -> Switch1/2
  Constant3/1 -> Switch1/1
  Switch3/1 -> Add/4
  Data Store Read4/1 -> Switch2/2
  Switch2/1 -> Add/3
  Data Store Read/1 -> Switch3/2
  Constant4/1 -> Switch1/3
  Switch/1 -> Add/1
  Constant5/1 -> Switch2/1
  Switch1/1 -> Add/2
  Constant7/1 -> Switch3/1
  Data Store Read6/1 -> Switch/2
  Add/1 -> Data Type Conversion1/1
  Constant1/1 -> Switch/1
  Constant2/1 -> Switch/3

== system VehCtrl20260630_18B/SigOut/GPIO /SPI3: LS03_06_07_08_10_12_13_17_18_19/Subsystem/控制 ==
  note: out1
  note: out2
  note: out3
  note: out5
  note: out4
  note: out7
  note: out6
  note: out8
  Add : Sum  Inputs=++++++++
  Add1 : Sum  Inputs=+++
  Constant1 : Constant  Value=0
  Constant2 : Constant  Value=0
  Constant9 : Constant  Value=44  OutDataTypeStr=uint8
  Data Store Read : DataStoreRead  DataStoreName=LS019
  Data Store Read1 : DataStoreRead  DataStoreName=LS007
  Data Store Read10 : DataStoreRead  DataStoreName=LS006
  Data Store Read2 : DataStoreRead  DataStoreName=LS012
  Data Store Read4 : DataStoreRead  DataStoreName=LS018
  Data Store Read5 : DataStoreRead  DataStoreName=LS010
  Data Store Read6 : DataStoreRead  DataStoreName=LS008
  Data Store Read7 : DataStoreRead  DataStoreName=LS003
  Data Store Read8 : DataStoreRead  DataStoreName=LS017
  Data Store Read9 : DataStoreRead  DataStoreName=LS013
  Data Type Conversion : DataTypeConversion  OutDataTypeStr=uint8
  Data Type Conversion1 : DataTypeConversion  OutDataTypeStr=uint8
  Gain : Gain
  Gain1 : Gain  Gain=2
  Gain2 : Gain  Gain=4
  Gain3 : Gain  Gain=8
  Gain4 : Gain  Gain=16
  Gain5 : Gain  Gain=32
  Gain6 : Gain  Gain=64
  Gain7 : Gain  Gain=128
  Gain8 : Gain
  Gain9 : Gain  Gain=2
  Terminator{,1..3} (4 alike) : Terminator
  Out1 : Outport  VectorParamsAs1DForOutWhenUnconnected=on
  Out2 : Outport  Port=2  VectorParamsAs1DForOutWhenUnconnected=on
  wires:
  Constant9/1 -> Add1/1
  Data Store Read10/1 -> Gain7/1
  Data Type Conversion1/1 -> Out2/1
  Data Store Read2/1 -> Gain9/1
  Add1/1 -> Data Type Conversion/1
  Add/1 -> Data Type Conversion1/1
  Data Store Read5/1 -> Gain2/1
  Gain6/1 -> Add/2
  Data Store Read1/1 -> Gain8/1
  Gain9/1 -> Add1/2
  Gain7/1 -> Add/1
  Gain/1 -> Add/8
  Data Type Conversion/1 -> Out1/1
  Data Store Read9/1 -> Gain6/1
  Gain4/1 -> Add/4
  Gain8/1 -> Add1/3
  Gain1/1 -> Add/7
  Data Store Read6/1 -> Gain3/1
  Gain3/1 -> Add/5
  Gain2/1 -> Add/6
  Gain5/1 -> Add/3
  Data Store Read8/1 -> Terminator/1
  Data Store Read7/1 -> Terminator1/1
  Constant1/1 -> Gain4/1, Gain5/1
  Data Store Read/1 -> Terminator3/1
  Data Store Read4/1 -> Terminator2/1
  Constant2/1 -> Gain/1, Gain1/1

== system VehCtrl20260630_18B/VehCtrl/MontionControl/DriveControl/Motor/Subsystem ==
  TmCtrMode : Inport
  TrqCmdRMT : Inport  Port=2
  Bus Selector3 : BusSelector  OutputSignals=Auto.signal3.AUTO_TrqCmdFL,EN,AutoMode
  Compare To Constant : simulink/Logic and Bit Operations/Compare To Constant  relop===  const=1  OutDataTypeStr=boolean
  Constant : Constant  Value=0
  Data Store Read : DataStoreRead  DataStoreName=CtrMode
  Data Type Conversion : DataTypeConversion
  Switch1 : Switch  Criteria=u2 > Threshold
  Switch3 : Switch  Criteria=u2 > Threshold
  Terminator : Terminator
  Out1 : Outport
  wires:
  Switch3/1 -> Out1/1
  TmCtrMode/1 -> Bus Selector3/1
  Bus Selector3/1 -> [TrqCmd]  "<AUTO_TrqCmdFL>"
  Bus Selector3/2 -> [EN]  "<EN>"
  Bus Selector3/3 -> [AutoMode]  "<AutoMode>"
  TrqCmdRMT/1 -> Switch1/3  "TrqCmdFL_RMT"
  [TrqCmd] -> Switch1/1  "TrqCmdFL_Auto"
  [EN] -> Switch3/2
  Constant/1 -> Data Type Conversion/1
  Switch1/1 -> Switch3/1  "TrqCtrFL"
  Compare To Constant/1 -> Switch1/2
  Data Store Read/1 -> Compare To Constant/1
  [AutoMode] -> Terminator/1
  Data Type Conversion/1 -> Switch3/3

== system VehCtrl20260630_18B/VehCtrl/MontionControl/DriveControl/Motor/Subsystem1 ==
  TmCtrMode : Inport
  TrqCmdRMT : Inport  Port=2
  Bus Selector3 : BusSelector  OutputSignals=Auto.signal3.AUTO_TrqCmdFR,EN,AutoMode
  Compare To Constant : simulink/Logic and Bit Operations/Compare To Constant  relop===  const=1  OutDataTypeStr=boolean
  Constant : Constant  Value=0
  Data Store Read : DataStoreRead  DataStoreName=CtrMode
  Data Type Conversion : DataTypeConversion
  Switch1 : Switch  Criteria=u2 > Threshold
  Switch3 : Switch  Criteria=u2 > Threshold
  Terminator : Terminator
  Out1 : Outport
  wires:
  Switch1/1 -> Switch3/1
  Constant/1 -> Data Type Conversion/1
  [EN] -> Switch3/2
  [TrqCmd] -> Switch1/1
  TrqCmdRMT/1 -> Switch1/3
  Compare To Constant/1 -> Switch1/2
  Bus Selector3/3 -> [AutoMode]  "<AutoMode>"
  Bus Selector3/2 -> [EN]  "<EN>"
  Bus Selector3/1 -> [TrqCmd]  "<AUTO_TrqCmdFR>"
  TmCtrMode/1 -> Bus Selector3/1
  Switch3/1 -> Out1/1
  Data Store Read/1 -> Compare To Constant/1
  [AutoMode] -> Terminator/1
  Data Type Conversion/1 -> Switch3/3

== system VehCtrl20260630_18B/VehCtrl/MontionControl/DriveControl/Motor/Subsystem2 ==
  TmCtrMode : Inport
  TrqCmdRMT : Inport  Port=2
  Bus Selector3 : BusSelector  OutputSignals=Auto.signal3.AUTO_TrqCmdRL,EN,AutoMode
  Compare To Constant : simulink/Logic and Bit Operations/Compare To Constant  relop===  const=1  OutDataTypeStr=boolean
  Constant : Constant  Value=0
  Data Store Read : DataStoreRead  DataStoreName=CtrMode
  Data Type Conversion : DataTypeConversion
  Switch1 : Switch  Criteria=u2 > Threshold
  Switch3 : Switch  Criteria=u2 > Threshold
  Terminator : Terminator
  Out1 : Outport
  wires:
  Switch3/1 -> Out1/1
  TmCtrMode/1 -> Bus Selector3/1
  Bus Selector3/1 -> [TrqCmd]  "<AUTO_TrqCmdRL>"
  Bus Selector3/2 -> [EN]  "<EN>"
  Bus Selector3/3 -> [AutoMode]  "<AutoMode>"
  Compare To Constant/1 -> Switch1/2
  TrqCmdRMT/1 -> Switch1/3
  [TrqCmd] -> Switch1/1
  [EN] -> Switch3/2
  Constant/1 -> Data Type Conversion/1
  Switch1/1 -> Switch3/1
  Data Store Read/1 -> Compare To Constant/1
  [AutoMode] -> Terminator/1
  Data Type Conversion/1 -> Switch3/3

== system VehCtrl20260630_18B/VehCtrl/MontionControl/DriveControl/Motor/Subsystem3 ==
  TmCtrMode : Inport
  TrqCmdRMT : Inport  Port=2
  Bus Selector3 : BusSelector  OutputSignals=Auto.signal3.AUTO_TrqCmdRR,EN,AutoMode
  Compare To Constant : simulink/Logic and Bit Operations/Compare To Constant  relop===  const=1  OutDataTypeStr=boolean
  Constant : Constant  Value=0
  Data Store Read : DataStoreRead  DataStoreName=CtrMode
  Data Type Conversion : DataTypeConversion
  Switch1 : Switch  Criteria=u2 > Threshold
  Switch3 : Switch  Criteria=u2 > Threshold
  Terminator : Terminator
  Out1 : Outport
  wires:
  Switch1/1 -> Switch3/1
  Constant/1 -> Data Type Conversion/1
  [EN] -> Switch3/2
  [TrqCmd] -> Switch1/1
  TrqCmdRMT/1 -> Switch1/3
  Compare To Constant/1 -> Switch1/2
  Bus Selector3/3 -> [AutoMode]  "<AutoMode>"
  Bus Selector3/2 -> [EN]  "<EN>"
  Bus Selector3/1 -> [TrqCmd]  "<AUTO_TrqCmdRR>"
  TmCtrMode/1 -> Bus Selector3/1
  Switch3/1 -> Out1/1
  Data Store Read/1 -> Compare To Constant/1
  [AutoMode] -> Terminator/1
  Data Type Conversion/1 -> Switch3/3

== system VehCtrl20260630_18B/VehCtrl/MontionControl/DriveControl/Motor/VehicleControl ==
  DrvPhase : Inport
  VehSpd [m/s] : Inport  Port=2
  VehDrvPct : Inport  Port=3
  PwrLim : Inport  Port=4
  RMT : Inport  Port=5
  Bus Selector1 : BusSelector  OutputSignals=RMT2.RMT_MtrTqGr
  Constant1 : Constant  Value=DRV_BACKWARD
  Constant2 : Constant  Value=DRV_FORWARD
  Constant3 : Constant  Value=0.0  OutDataTypeStr=single
  GreaterThan1 : RelationalOperator  Operator===  OutDataTypeStr=boolean  RndMeth=Simplest
  GreaterThan2 : RelationalOperator  Operator===  OutDataTypeStr=boolean  RndMeth=Simplest
  Product : Product
  Switch1 : Switch  Criteria=u2 > Threshold
  Switch2 : Switch  Criteria=u2 > Threshold
  VehTrqBackward : Subsystem
  VehTrqForward : Subsystem
  VehTrq [Nm] : Outport
  wires:
  DrvPhase/1 -> GreaterThan2/1, GreaterThan1/1
  Switch1/1 -> Product/1  "VehTrq"
  Constant1/1 -> GreaterThan1/2
  GreaterThan1/1 -> Switch1/2
  Switch2/1 -> Switch1/3
  Constant2/1 -> GreaterThan2/2
  GreaterThan2/1 -> Switch2/2
  VehTrqBackward/1(VehTrq) -> Switch1/1
  VehTrqForward/1(VehTrq) -> Switch2/1
  Constant3/1 -> Switch2/3
  VehDrvPct/1 -> VehTrqForward/2(VehDrv), VehTrqBackward/2(VehDrvPct)
  VehSpd [m/s]/1 -> VehTrqForward/1(VehSpd), VehTrqBackward/1(VehSpd)
  PwrLim/1 -> VehTrqForward/3(PwrLim), VehTrqBackward/3(PwrLim)
  RMT/1 -> Bus Selector1/1
  Bus Selector1/1 -> Product/2  "<RMT_MtrTqGr>"
  Product/1 -> VehTrq [Nm]/1  "VehTrq_ter"

== system VehCtrl20260630_18B/VehCtrl/MontionControl/DriveControl/Motor/WheelControl ==
  DrvPhase : Inport
  VehTrq : Inport  Port=2
  CmdStrAng : Inport  Port=3
  Chart : Stateflow chart  TreatAsAtomicUnit=on
  Constant : Constant  Value=MtrTrqMax
  Data Store Read : DataStoreRead  DataStoreName=MtrTrqZeroturn
  Data Store Read1 : DataStoreRead  DataStoreName=FacFrontInter
  Data Store Read2 : DataStoreRead  DataStoreName=FacFrontOuter
  Data Store Read3 : DataStoreRead  DataStoreName=FacRearInter
  Data Store Read4 : DataStoreRead  DataStoreName=FacRearOuter
  MtrDirCmdFL : Outport
  MtrDirCmdFR : Outport  Port=2
  MtrDirCmdRL : Outport  Port=3
  MtrDirCmdRR : Outport  Port=4
  MtrTrqCmdFL : Outport  Port=5
  MtrTrqCmdFR : Outport  Port=6
  MtrTrqCmdRL : Outport  Port=7
  MtrTrqCmdRR : Outport  Port=8
  wires:
  Chart/5(MtrTrqCmdFL) -> MtrTrqCmdFL/1
  Chart/4(MtrDirCmdRR) -> MtrDirCmdRR/1  "MtrDirCmdRR"
  VehTrq/1 -> Chart/2(VehTrq)
  Chart/2(MtrDirCmdFR) -> MtrDirCmdFR/1  "MtrDirCmdFR"
  Chart/8(MtrTrqCmdRR) -> MtrTrqCmdRR/1
  Chart/6(MtrTrqCmdFR) -> MtrTrqCmdFR/1
  Chart/7(MtrTrqCmdRL) -> MtrTrqCmdRL/1
  Chart/1(MtrDirCmdFL) -> MtrDirCmdFL/1  "MtrDirCmdFL"
  CmdStrAng/1 -> Chart/4(CmdStrAng)
  Chart/3(MtrDirCmdRL) -> MtrDirCmdRL/1  "MtrDirCmdRL"
  DrvPhase/1 -> Chart/1(DrvPhase)
  Data Store Read/1 -> Chart/5(MtrTrqZeroturn)
  Data Store Read1/1 -> Chart/6(FacFrontInter)
  Data Store Read2/1 -> Chart/7(FacFrontOuter)
  Data Store Read4/1 -> Chart/9(FacRearOuter)
  Data Store Read3/1 -> Chart/8(FacRearInter)
  Constant/1 -> Chart/3(TrqMax)

== system VehCtrl20260630_18B/VehCtrl/MontionControl/ValveControl/SteerSys/Controller ==
  In1 : Inport
  In2 : Inport  Port=2
  In3 : Inport  Port=3
  1-D Lookup Table : Lookup_n-D  NumberOfTableDimensions=1  BreakpointsForDimension1=VehSpd  Table=Kp1  InternalRulePriority=Speed  RndMeth=Simplest  InputSameDT=on
  1-D Lookup Table1 : Lookup_n-D  NumberOfTableDimensions=1  BreakpointsForDimension1=VehSpd  Table=Kp2  InternalRulePriority=Speed  RndMeth=Simplest  InputSameDT=on
  Abs : Abs
  Add : Sum
  Data Store Read : DataStoreRead  DataStoreName=Kd
  Data Type Conversion : DataTypeConversion  OutDataTypeStr=double
  Data Type Conversion1 : DataTypeConversion  OutDataTypeStr=single
  Data Type Conversion2 : DataTypeConversion  OutDataTypeStr=double
  Dead Zone : DeadZone  LowerValue=-15  UpperValue=15  SaturateOnIntegerOverflow=on
  Derivative2 : Derivative
  Product : Product
  Product1 : Product
  Saturation : Saturate  UpperLimit=100  LowerLimit=-100
  Saturation1 : Saturate  UpperLimit=36  LowerLimit=18
  Switch : Switch  Criteria=u2 > Threshold
  Out1 : Outport
  wires:
  Data Type Conversion1/1 -> Saturation/1
  Saturation/1 -> Dead Zone/1
  Saturation1/1 -> Product/2  "kp"
  In1/1 -> Data Type Conversion/1
  Abs/1 -> Out1/1
  Dead Zone/1 -> Abs/1
  In2/1 -> Data Type Conversion2/1
  Data Type Conversion2/1 -> 1-D Lookup Table1/1, 1-D Lookup Table/1
  1-D Lookup Table/1 -> Switch/1
  Data Type Conversion/1 -> Product1/2, Product/1
  Derivative2/1 -> Add/1
  Product1/1 -> Derivative2/1
  Data Store Read/1 -> Product1/1
  Add/1 -> Data Type Conversion1/1
  Product/1 -> Add/2
  In3/1 -> Switch/2
  1-D Lookup Table1/1 -> Switch/3
  Switch/1 -> Saturation1/1

== system VehCtrl20260630_18B/VehCtrl/MontionControl/ValveControl/SteerSys/LEFT ==
  note: 左正右负，左转限制左边幅值
  "SteerFL " : Inport
  In1 : Inport  Port=2
  SteerFR : Inport  Port=3
  Action Port : ActionPort  ActionType=then
  Add1 : Sum  Inputs=-+
  Add4 : Sum  Inputs=-+
  Compare To Constant : simulink/Logic and Bit Operations/Compare To Constant  relop=>  const=0  OutDataTypeStr=boolean
  Compare To Constant1 : simulink/Logic and Bit Operations/Compare To Constant  relop=>  const=0  OutDataTypeStr=boolean
  Constant : Constant  Value=0  OutDataTypeStr=single
  Constant1 : Constant  Value=SteerAngMax
  Constant2 : Constant
  Constant3 : Constant  Value=0
  Constant6 : Constant  Value=SteerAngMax
  Data Type Conversion : DataTypeConversion
  Logical Operator : Logic  Operator=OR  AllPortsSameDT=off  OutDataTypeStr=boolean
  Mux : Mux  Inputs=2
  Product2 : Product
  Switch1 : Switch  Criteria=u2 > Threshold
  Out1 : Outport
  wires:
  Constant/1 -> Mux/2
  In1/1 -> Product2/2
  Mux/1 -> Out1/1
  Constant2/1 -> Switch1/3
  Constant3/1 -> Switch1/1
  Constant1/1 -> Add1/1
  Switch1/1 -> [SteerK]
  [SteerK] -> Product2/1
  Product2/1 -> Data Type Conversion/1
  Data Type Conversion/1 -> Mux/1
  Constant6/1 -> Add4/1
  Add1/1 -> Compare To Constant/1
  Add4/1 -> Compare To Constant1/1
  Logical Operator/1 -> Switch1/2
  Compare To Constant/1 -> Logical Operator/1
  Compare To Constant1/1 -> Logical Operator/2
  "SteerFL "/1 -> Add1/2
  SteerFR/1 -> Add4/2

== system VehCtrl20260630_18B/VehCtrl/MontionControl/ValveControl/SteerSys/NATURAL  ==
  Action Port : ActionPort  ActionType=else
  Constant : Constant  Value=0  OutDataTypeStr=single
  Constant1 : Constant  Value=0  OutDataTypeStr=single
  Mux : Mux  Inputs=2
  Out1 : Outport
  wires:
  Constant/1 -> Mux/1
  Mux/1 -> Out1/1
  Constant1/1 -> Mux/2

== system VehCtrl20260630_18B/VehCtrl/MontionControl/ValveControl/SteerSys/RIGHT ==
  note: 左正右负，右转限制右边幅值
  SteerFL : Inport
  In1 : Inport  Port=2
  SteerFR : Inport  Port=3
  Action Port : ActionPort  ActionType=elseif
  Add3 : Sum  Inputs=-+
  Add6 : Sum  Inputs=-+
  Compare To Constant : simulink/Logic and Bit Operations/Compare To Constant  relop=>  const=0  OutDataTypeStr=boolean
  Compare To Constant1 : simulink/Logic and Bit Operations/Compare To Constant  relop=>  const=0  OutDataTypeStr=boolean
  Constant1 : Constant
  Constant2 : Constant  Value=0
  Constant4 : Constant  Value=0  OutDataTypeStr=single
  Constant5 : Constant  Value=SteerAngMax
  Constant8 : Constant  Value=SteerAngMax
  Data Type Conversion : DataTypeConversion
  Gain : Gain  Gain=-1
  Gain1 : Gain  Gain=-1
  Logical Operator : Logic  Operator=OR  AllPortsSameDT=off  OutDataTypeStr=boolean
  Mux : Mux  Inputs=2
  Product1 : Product
  Switch1 : Switch  Criteria=u2 > Threshold
  Out1 : Outport
  wires:
  Mux/1 -> Out1/1
  Constant4/1 -> Mux/1
  Constant1/1 -> Switch1/3
  Constant2/1 -> Switch1/1
  Switch1/1 -> [SteerK]
  Logical Operator/1 -> Switch1/2
  [SteerK] -> Product1/2
  In1/1 -> Product1/1
  Product1/1 -> Data Type Conversion/1
  Data Type Conversion/1 -> Mux/2
  Constant5/1 -> Add3/1
  Compare To Constant1/1 -> Logical Operator/2
  Compare To Constant/1 -> Logical Operator/1
  Add6/1 -> Compare To Constant1/1
  Constant8/1 -> Add6/1
  Add3/1 -> Compare To Constant/1
  Gain/1 -> Add3/2
  Gain1/1 -> Add6/2
  SteerFL/1 -> Gain/1
  SteerFR/1 -> Gain1/1

== system VehCtrl20260630_18B/VehCtrl/MontionControl/ValveControl/SteerSys/Subsystem ==
  In1 : Inport
  Abs1 : Abs
  If1 : If  ElseIfExpressions=u1 < 0
  LEFT1 : Subsystem  TreatAsAtomicUnit=on
  Merge1 : Merge  Inputs=3
  NATURAL 1 : Subsystem  TreatAsAtomicUnit=on
  RIGHT1 : Subsystem  TreatAsAtomicUnit=on
  Out1 : Outport
  wires:
  LEFT1/1(Out1) -> Merge1/1
  In1/1 -> If1/1, Abs1/1
  Abs1/1 -> RIGHT1/1(In1), LEFT1/1(In1)
  NATURAL 1/1(Out1) -> Merge1/3
  If1/3 -> NATURAL 1/Action
  If1/2 -> RIGHT1/Action
  RIGHT1/1(Out1) -> Merge1/2
  If1/1 -> LEFT1/Action
  Merge1/1 -> Out1/1

== system VehCtrl20260630_18B/VehCtrl/MontionControl/ValveControl/SteerSys/Subsystem1 ==
  SteerFL : Inport
  In2 : Inport  Port=2
  "SteerFR " : Inport  Port=3
  Add : Sum
  Product : Product
  Out1 : Outport
  wires:
  Add/1 -> Product/1
  Product/1 -> Out1/1
  SteerFL/1 -> Add/1
  "SteerFR "/1 -> Add/2
  In2/1 -> Product/2

== system VehCtrl20260630_18B/VehCtrl/MontionControl/DriveControl/Motor/VehicleControl/VehTrqBackward ==
  VehSpd : Inport
  VehDrvPct : Inport  Port=2
  PwrLim : Inport  Port=3
  Abs : Abs
  Constant : Constant  Value=VehTrqBackwardMax
  Constant1 : Constant  Value=VehPwrBackwardMax
  Constant2 : Constant  Value=WhlRadius
  Constant3 : Constant  Value=0.1  OutDataTypeStr=single
  Divide : Product  Inputs=*/
  Divide1 : Product  Inputs=*/
  Gain : Gain  Gain=1000
  Gain1 : Gain  Gain=0.01
  Gain2 : Gain  Gain=PwrLimFactor
  Max : MinMax  Function=max  Inputs=2
  Min : MinMax  Inputs=2
  Product : Product
  Product1 : Product
  Product2 : Product
  Switch : Switch  Criteria=u2 > Threshold
  VehTrq : Outport
  wires:
  VehDrvPct/1 -> Gain1/1
  Constant/1 -> Product1/2
  Product1/1 -> Min/1
  Gain1/1 -> Product/2, Product/1, Product1/1
  Product2/1 -> Divide/1
  Divide1/1 -> Divide/2
  Product/1 -> Product2/1
  Divide/1 -> Min/2
  Min/1 -> VehTrq/1
  Constant2/1 -> Divide1/2
  Constant3/1 -> Max/2
  Max/1 -> Divide1/1
  VehSpd/1 -> Abs/1
  Abs/1 -> Max/1
  Switch/1 -> Product2/2
  Constant1/1 -> Gain/1
  PwrLim/1 -> Switch/2
  Gain2/1 -> Switch/1
  Gain/1 -> Switch/3, Gain2/1
